simulink model "isi"  (Simulink 7.0)
settings: Solver=ode45  StartTime=0.0  StopTime=10.0  RelTol=1e-3
libraries: cdsFilt x103, cdsEpicsBinIn x13, cdsEpicsOut x12, cdsMuxMatrix x4, cdsEpicsIn x3, cdsWD x3, cdsRio x2, cdsMatrix x2, dac x1, cdsSwitch x1, cdsParameters x1
(part 5 of 7)

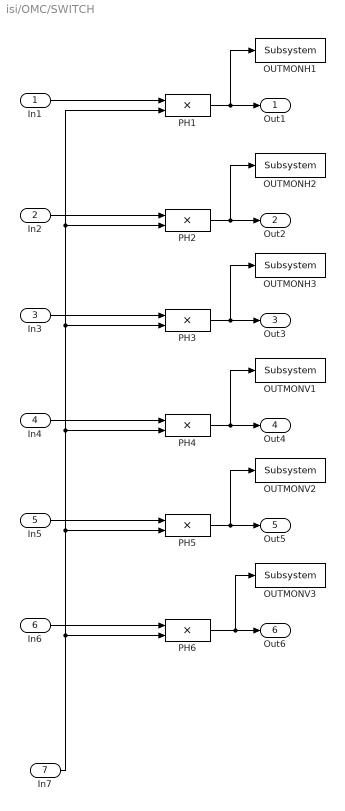
== system isi/OMC/SWITCH ==
  In1 : Inport  OutDataType=sfix(16)  OutScaling=2^0
  In2 : Inport  Port=2  OutDataType=sfix(16)  OutScaling=2^0
  In3 : Inport  Port=3  OutDataType=sfix(16)  OutScaling=2^0
  In4 : Inport  Port=4  OutDataType=sfix(16)  OutScaling=2^0
  In5 : Inport  Port=5  OutDataType=sfix(16)  OutScaling=2^0
  In6 : Inport  Port=6  OutDataType=sfix(16)  OutScaling=2^0
  In7 : Inport  Port=7  OutDataType=sfix(16)  OutScaling=2^0
  OUTMONH1 : cdsFilt/Subsystem  Tag=cdsFilt  Description=|  SystemSampleTime=-1
      | Purpose:                                                                                                                                                                                                                                  
      | Standard CDS IIR filter module.                                                                                                                                                                                                           
      |                                                                                                                                                                                                                                           
      | Operation:                                                                                                                                                                                                                                
      | Consists of 10 second order section IIR filters, plus a ramped gain stage. In FE code, also provides pre-defined test points and excitation channel inputs. The filter coefficients are defined in the LIGO system using the 'foton' tool.
      |                                                                                                                                                                                                                                           
      | Usage:                                                                                                                                                                                                                                    
      | Name the part with the desired filter module name.
      settings: AttributesFormatString=%<Tag>
  OUTMONH2 : cdsFilt/Subsystem  Tag=cdsFilt  Description=|  SystemSampleTime=-1
      | Purpose:                                                                                                                                                                                                                                  
      | Standard CDS IIR filter module.                                                                                                                                                                                                           
      |                                                                                                                                                                                                                                           
      | Operation:                                                                                                                                                                                                                                
      | Consists of 10 second order section IIR filters, plus a ramped gain stage. In FE code, also provides pre-defined test points and excitation channel inputs. The filter coefficients are defined in the LIGO system using the 'foton' tool.
      |                                                                                                                                                                                                                                           
      | Usage:                                                                                                                                                                                                                                    
      | Name the part with the desired filter module name.
      settings: AttributesFormatString=%<Tag>
  OUTMONH3 : cdsFilt/Subsystem  Tag=cdsFilt  Description=|  SystemSampleTime=-1
      | Purpose:                                                                                                                                                                                                                                  
      | Standard CDS IIR filter module.                                                                                                                                                                                                           
      |                                                                                                                                                                                                                                           
      | Operation:                                                                                                                                                                                                                                
      | Consists of 10 second order section IIR filters, plus a ramped gain stage. In FE code, also provides pre-defined test points and excitation channel inputs. The filter coefficients are defined in the LIGO system using the 'foton' tool.
      |                                                                                                                                                                                                                                           
      | Usage:                                                                                                                                                                                                                                    
      | Name the part with the desired filter module name.
      settings: AttributesFormatString=%<Tag>
  OUTMONV1 : cdsFilt/Subsystem  Tag=cdsFilt  Description=|  SystemSampleTime=-1
      | Purpose:                                                                                                                                                                                                                                  
      | Standard CDS IIR filter module.                                                                                                                                                                                                           
      |                                                                                                                                                                                                                                           
      | Operation:                                                                                                                                                                                                                                
      | Consists of 10 second order section IIR filters, plus a ramped gain stage. In FE code, also provides pre-defined test points and excitation channel inputs. The filter coefficients are defined in the LIGO system using the 'foton' tool.
      |                                                                                                                                                                                                                                           
      | Usage:                                                                                                                                                                                                                                    
      | Name the part with the desired filter module name.
      settings: AttributesFormatString=%<Tag>
  OUTMONV2 : cdsFilt/Subsystem  Tag=cdsFilt  Description=|  SystemSampleTime=-1
      | Purpose:                                                                                                                                                                                                                                  
      | Standard CDS IIR filter module.                                                                                                                                                                                                           
      |                                                                                                                                                                                                                                           
      | Operation:                                                                                                                                                                                                                                
      | Consists of 10 second order section IIR filters, plus a ramped gain stage. In FE code, also provides pre-defined test points and excitation channel inputs. The filter coefficients are defined in the LIGO system using the 'foton' tool.
      |                                                                                                                                                                                                                                           
      | Usage:                                                                                                                                                                                                                                    
      | Name the part with the desired filter module name.
      settings: AttributesFormatString=%<Tag>
  OUTMONV3 : cdsFilt/Subsystem  Tag=cdsFilt  Description=|  SystemSampleTime=-1
      | Purpose:                                                                                                                                                                                                                                  
      | Standard CDS IIR filter module.                                                                                                                                                                                                           
      |                                                                                                                                                                                                                                           
      | Operation:                                                                                                                                                                                                                                
      | Consists of 10 second order section IIR filters, plus a ramped gain stage. In FE code, also provides pre-defined test points and excitation channel inputs. The filter coefficients are defined in the LIGO system using the 'foton' tool.
      |                                                                                                                                                                                                                                           
      | Usage:                                                                                                                                                                                                                                    
      | Name the part with the desired filter module name.
      settings: AttributesFormatString=%<Tag>
  PH{1..6} (6 alike) : Product  OutDataType=sfix(16)  OutScaling=2^0  RndMeth=Zero
  Out1 : Outport  OutDataType=sfix(16)  OutScaling=2^0
  Out2 : Outport  Port=2  OutDataType=sfix(16)  OutScaling=2^0
  Out3 : Outport  Port=3  OutDataType=sfix(16)  OutScaling=2^0
  Out4 : Outport  Port=4  OutDataType=sfix(16)  OutScaling=2^0
  Out5 : Outport  Port=5  OutDataType=sfix(16)  OutScaling=2^0
  Out6 : Outport  Port=6  OutDataType=sfix(16)  OutScaling=2^0
  wires:
  In6/1 -> PH6/1
  In5/1 -> PH5/1
  In4/1 -> PH4/1
  In3/1 -> PH3/1
  In2/1 -> PH2/1
  PH6/1 -> Out6/1, OUTMONV3/1
  PH5/1 -> Out5/1, OUTMONV2/1
  PH4/1 -> Out4/1, OUTMONV1/1
  PH3/1 -> Out3/1, OUTMONH3/1
  PH2/1 -> Out2/1, OUTMONH2/1
  In7/1 -> PH6/2, PH5/2, PH4/2, PH3/2, PH2/2, PH1/2
  PH1/1 -> Out1/1, OUTMONH1/1
  In1/1 -> PH1/1

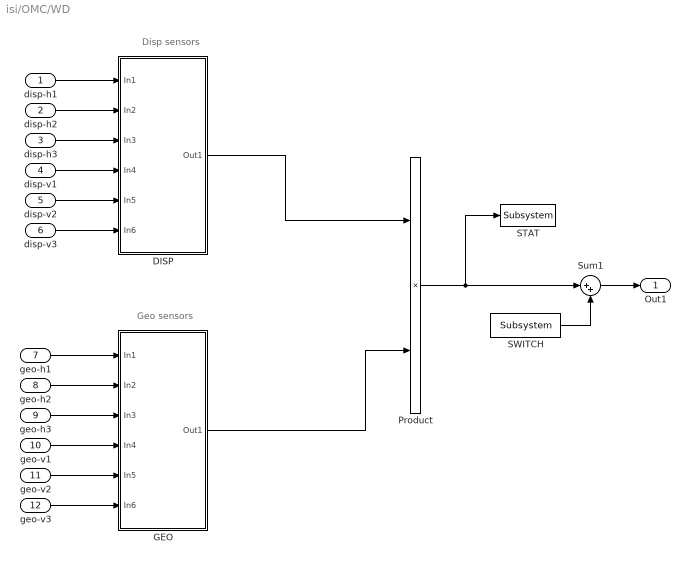
== system isi/OMC/WD ==
  note: Disp sensors
  note: Geo sensors
  disp-h1 : Inport  OutDataType=sfix(16)  OutScaling=2^0
  disp-h2 : Inport  Port=2  OutDataType=sfix(16)  OutScaling=2^0
  disp-h3 : Inport  Port=3  OutDataType=sfix(16)  OutScaling=2^0
  disp-v1 : Inport  Port=4  OutDataType=sfix(16)  OutScaling=2^0
  disp-v2 : Inport  Port=5  OutDataType=sfix(16)  OutScaling=2^0
  disp-v3 : Inport  Port=6  OutDataType=sfix(16)  OutScaling=2^0
  geo-h1 : Inport  Port=7  OutDataType=sfix(16)  OutScaling=2^0
  geo-h2 : Inport  Port=8  OutDataType=sfix(16)  OutScaling=2^0
  geo-h3 : Inport  Port=9  OutDataType=sfix(16)  OutScaling=2^0
  geo-v1 : Inport  Port=10  OutDataType=sfix(16)  OutScaling=2^0
  geo-v2 : Inport  Port=11  OutDataType=sfix(16)  OutScaling=2^0
  geo-v3 : Inport  Port=12  OutDataType=sfix(16)  OutScaling=2^0
  DISP : Subsystem
  GEO : Subsystem
  Product : Product  OutDataType=sfix(16)  OutScaling=2^0  RndMeth=Zero
  STAT : cdsEpicsOut/Subsystem  Tag=cdsEpicsOutput  Description=|  SystemSampleTime=-1
      | Purpose:                                          
      | Output a FE signal to an EPICS channel.           
      |                                                   
      | Operation:                                        
      | Takes input value and passes it to EPICS record.  
      |                                                   
      | Usage:                                            
      | Name the part with the desired EPICS rrecord name.
      settings: AttributesFormatString=%<Tag>
  SWITCH : cdsEpicsIn/Subsystem  Tag=cdsEpicsIn  Description=|  SystemSampleTime=-1
      | Purpose:                                                                              
      | Create an EPICS input channel connection to the FE realtime controls.                 
      |                                                                                       
      | Operation:                                                                            
      | Outputs value from an EPICS ai record. Value is floating point with a precision of 3..
      |                                                                                       
      | Usage:                                                                                
      | Name the part with the desired EPICS channel name.
      settings: AttributesFormatString=%<Tag>
  Sum1 : Sum  Inputs=|++  OutDataType=sfix(16)  OutScaling=2^0
  Out1 : Outport  OutDataType=sfix(16)  OutScaling=2^0
  wires:
  disp-h1/1 -> DISP/1(In1)
  disp-h2/1 -> DISP/2(In2)
  disp-h3/1 -> DISP/3(In3)
  disp-v1/1 -> DISP/4(In4)
  disp-v2/1 -> DISP/5(In5)
  disp-v3/1 -> DISP/6(In6)
  geo-h1/1 -> GEO/1(In1)
  geo-h2/1 -> GEO/2(In2)
  geo-h3/1 -> GEO/3(In3)
  geo-v1/1 -> GEO/4(In4)
  geo-v2/1 -> GEO/5(In5)
  geo-v3/1 -> GEO/6(In6)
  DISP/1(Out1) -> Product/1
  Product/1 -> STAT/1, Sum1/1
  GEO/1(Out1) -> Product/2
  Sum1/1 -> Out1/1
  SWITCH/1 -> Sum1/2
